simulink model "LinearizedTop"  (R2019a)
settings: Solver=FixedStepAuto  StartTime=0.0  StopTime=10  FixedStep=0.001  RelTol=1e-3
values from neighbouring files (symbols this model uses):
  Parameters = ConvertParams(X)    [EstimatedParams.m]    (also in LQR.m = EstimatedParams(); LSQnonLinfunc.m = CoenParams(X); TestModel.m = CoenParams(X0); testingLQRDisturbance.m = EstimatedParams())
settings Model: Creator=houte  LastModifiedBy=coeng

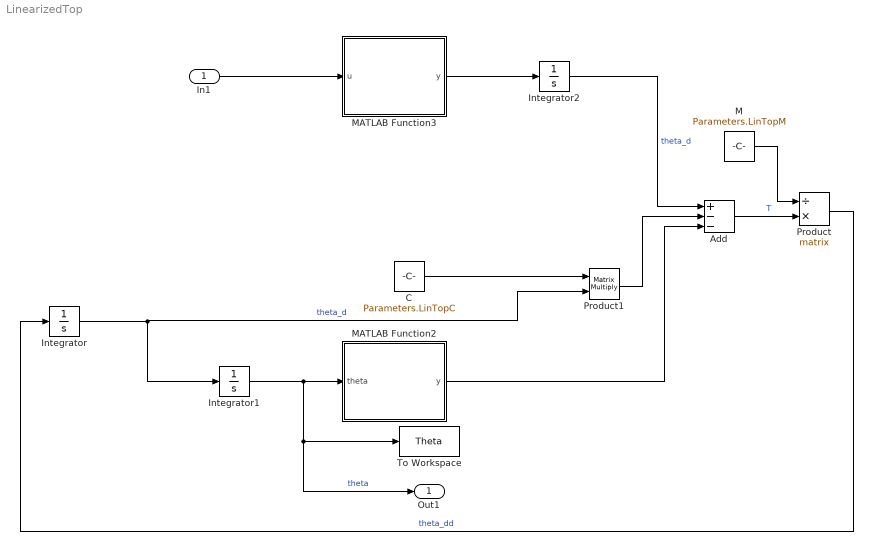
== system LinearizedTop ==
  In1 : Inport
  Add : Sum  Inputs=+--
  C : Constant  Value=Parameters.LinTopC
  Integrator : Integrator  InitialCondition=[0; 0]
  Integrator1 : Integrator  InitialCondition=firstLocation'
  Integrator2 : Integrator  InitialCondition=[0; 0]
  "M " : Constant  Value=Parameters.LinTopM
  MATLAB Function2 : MATLAB Function  TreatAsAtomicUnit=on
  MATLAB Function3 : MATLAB Function  TreatAsAtomicUnit=on
  Product : Product  Inputs=/*  Multiplication=Matrix(*)
  Product1 : Product  Multiplication=Matrix(*)
  To Workspace : ToWorkspace  VariableName=Theta  SaveFormat=Timeseries  SampleTime=-1
  Out1 : Outport
  wires:
  Integrator/1 -> Product1/2, Integrator1/1  "theta_d"
  Integrator1/1 -> Out1/1, To Workspace/1, MATLAB Function2/1(theta)  "theta"
  Add/1 -> Product/2  "T"
  MATLAB Function3/1(y) -> Integrator2/1
  MATLAB Function2/1(y) -> Add/3
  Product/1 -> Integrator/1  "theta_dd"
  Integrator2/1 -> Add/1  "theta_d"
  Product1/1 -> Add/2
  In1/1 -> MATLAB Function3/1(u)
  C/1 -> Product1/1
  "M "/1 -> Product/1

== matlab function LinearizedTop/MATLAB Function2 ==
  data: theta input; y output; Parameters parameter
function y = G(theta, Parameters)
    theta1 = theta(1);
    theta2 = theta(2);

y = [-Parameters.g1*theta1 - Parameters.g2*(-theta2 + pi - theta1);
     -Parameters.g2*(-theta2 + pi - theta1)]

== matlab function LinearizedTop/MATLAB Function3 ==
  data: u input; y output; Parameters parameter
function y = T(u, Parameters)
    % T = km*u - Te*dTe;
    %dTe = (km*u-T)/Te
    dTe = (Parameters.km*u-T(1))/Parameters.Te;
y = [dTe; 0];
